simulink model "solar_phto"  (R2025b)
settings: Solver=VariableStepAuto  StartTime=0.0  StopTime=10.0  RelTol=1e-3
InitFcn:
  | v=26.3
  | I=7.61
  | Iscn=8.21
  | Voc=32.9
  | Ipv=8.214
  | a=1.2;
  | Rp=415.405
  | Rs=0.221
  | Kv=0.1230
  | Ki=0.0032
  | Ipvn=8.214
  | Tn=300
  | Gn=1000
  | q=1.6*10^-19
  | k=1.38*10^-23
  | Ns=54
  | Ion=9.825*10^-8
  | Nser=26
  | Npar=5
libraries: spsSeriesRLCBranchLib x2, spsControlledCurrentSourceLib x1, spsCurrentMeasurementLib x1, spsVoltageMeasurementLib x1
settings Model: Creator=hp  LastModifiedBy=hp

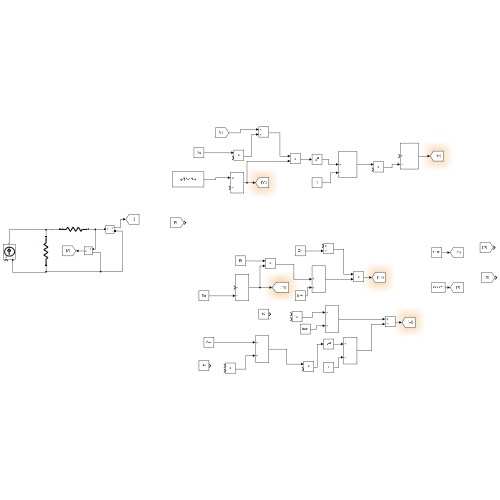
[thumbnail: Simulink's stored preview of the top-level diagram]
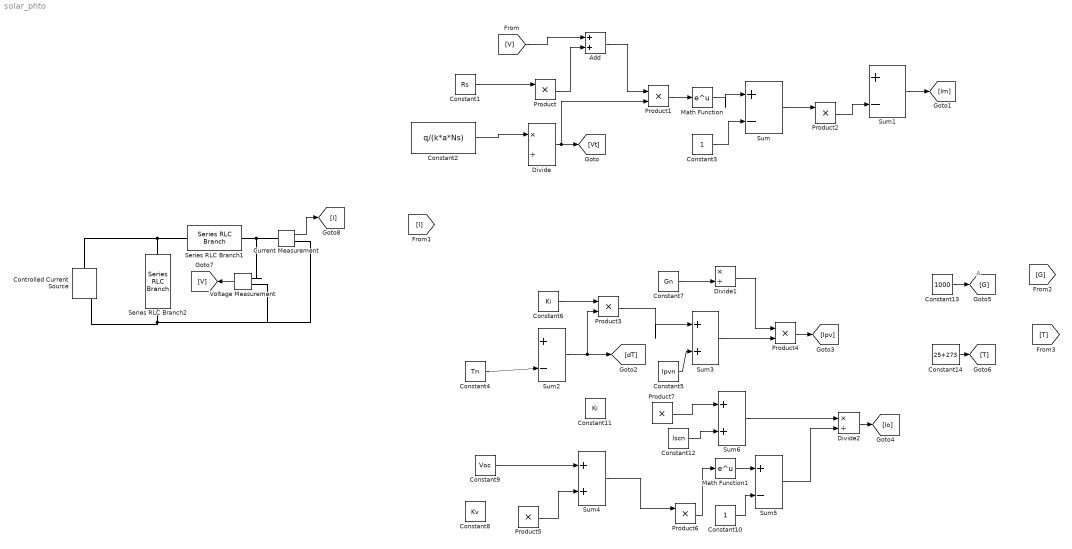
== system solar_phto ==
  note: A
  Add : Sum
  Constant1 : Constant  Value=Rs
  Constant10 : Constant
  Constant11 : Constant  Value=Ki
  Constant12 : Constant  Value=Iscn
  Constant13 : Constant  Value=1000
  Constant14 : Constant  Value=25+273
  Constant2 : Constant  Value=q/(k*a*Ns)
  Constant3 : Constant
  Constant4 : Constant  Value=Tn
  Constant5 : Constant  Value=Ipvn  VectorParams1D=off
  Constant6 : Constant  Value=Ki
  Constant7 : Constant  Value=Gn
  Constant8 : Constant  Value=Kv
  Constant9 : Constant  Value=Voc
  Controlled Current Source : spsControlledCurrentSourceLib/Controlled Current Source  Initialize=on  Source_Type=DC  Amplitude=0  Phase=0  Frequency=0  Measurements=None
  Current Measurement : spsCurrentMeasurementLib/Current Measurement  PhasorSimulation=off  OutputType=Complex  PSBequivalent=0
  Divide : Product  Inputs=*/
  Divide1 : Product  Inputs=*/
  Divide2 : Product  Inputs=*/
  Math Function : Math
  Math Function1 : Math
  Product{,1..7} (8 alike) : Product
  Series RLC Branch1 : spsSeriesRLCBranchLib/Series RLC Branch  LConnTagsString=__new0  RConnTagsString=__new0  BranchType=R  Resistance=Rs  Inductance=3e-3  SetiL0=off  InitialCurrent=0  Capacitance=1e-6  Setx0=off  InitialVoltage=0  Measurements=None
  Series RLC Branch2 : spsSeriesRLCBranchLib/Series RLC Branch  LConnTagsString=__new0  RConnTagsString=__new0  BranchType=R  Resistance=Rp  Inductance=3e-3  SetiL0=off  InitialCurrent=0  Capacitance=1e-6  Setx0=off  InitialVoltage=0  Measurements=None
  Sum : Sum  Inputs=|+-
  Sum1 : Sum  Inputs=|+-
  Sum2 : Sum  Inputs=|+-
  Sum3 : Sum  Inputs=|++
  Sum4 : Sum
  Sum5 : Sum  Inputs=+-
  Sum6 : Sum
  Voltage Measurement : spsVoltageMeasurementLib/Voltage Measurement  PhasorSimulation=off  OutputType=Complex  PSBequivalent=0
  wires:
  Constant1/1 -> Product/1
  Product/1 -> Add/2
  Add/1 -> Product1/1
  Constant2/1 -> Divide/1
  Divide/1 -> Product1/2, [Vt]
  Product1/1 -> Math Function/1
  Math Function/1 -> Sum/1
  Constant3/1 -> Sum/2
  Sum/1 -> Product2/1
  Product2/1 -> Sum1/2
  Sum1/1 -> [lm]
  Constant4/1 -> Sum2/2
  Constant6/1 -> Product3/1
  Sum2/1 -> Product3/2, [dT]
  Product3/1 -> Sum3/1
  Constant5/1 -> Sum3/2
  Constant7/1 -> Divide1/2
  Sum3/1 -> Product4/2
  Divide1/1 -> Product4/1
  Product4/1 -> [Ipv]
  Constant9/1 -> Sum4/1
  Product5/1 -> Sum4/2
  Sum4/1 -> Product6/1
  Product6/1 -> Math Function1/1
  Math Function1/1 -> Sum5/1
  Constant10/1 -> Sum5/2
  Product7/1 -> Sum6/1
  Constant12/1 -> Sum6/2
  Sum6/1 -> Divide2/1
  Sum5/1 -> Divide2/2
  Divide2/1 -> [lo]
  Constant13/1 -> [G]
  Constant14/1 -> [T]
  Voltage Measurement/1 -> [V]
  Current Measurement/1 -> [I]
  [V] -> Add/1
  connections:
  Series RLC Branch2/LConn1 -- Series RLC Branch1/LConn1 -- Controlled Current Source/RConn1
  Series RLC Branch2/RConn1 -- Current Measurement/RConn1 -- Voltage Measurement/LConn2 -- Controlled Current Source/LConn1
  Voltage Measurement/LConn1 -- Series RLC Branch1/RConn1 -- Current Measurement/LConn1
